simulink model "airplane_pitch_ctrl"  (R2014a)
settings: Solver=ode45  StartTime=0.0  StopTime=5  RelTol=1e-3
libraries: simulink x1
settings Model: Creator=Felix  LastModifiedBy=Felix

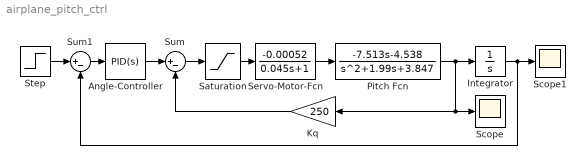
== system airplane_pitch_ctrl ==
  Angle-Controller : simulink/Continuous/PID Controller  Controller=PID  TimeDomain=Continuous-time  SampleTime=1  IntegratorMethod=Forward Euler  FilterMethod=Forward Euler  Form=Parallel  P=7000  I=200  D=1000  N=100  InitialConditionSource=internal  InitialConditionForIntegrator=0  InitialConditionForFilter=0  ExternalReset=none  LimitOutput=off  UpperSaturationLimit=inf  LowerSaturationLimit=-inf  LinearizeAsGain=on  AntiWindupMode=none  Kb=1  TrackingMode=off  Kt=1  PParamMin=[]  PParamMax=[]  PParamDataTypeStr=double  IParamMin=[]  IParamMax=[]  IParamDataTypeStr=double  DParamMin=[]  DParamMax=[]  NParamMin=[]  NParamMax=[]  KbParamMin=[]  KbParamMax=[]  KtParamMin=[]  KtParamMax=[]  POutMin=[]  POutMax=[]  POutDataTypeStr=double  IOutMin=[]  IOutMax=[]  IOutDataTypeStr=double  DOutMin=[]  DOutMax=[]  NOutMin=[]  NOutMax=[]  KbOutMin=[]  KbOutMax=[]  KtOutMin=[]  KtOutMax=[]  IntegratorOutMin=[]  IntegratorOutMax=[]  IntegratorOutDataTypeStr=single  FilterOutMin=[]  FilterOutMax=[]  SumOutMin=[]  SumOutMax=[]  SumOutDataTypeStr=double  SumI1OutMin=[]  SumI1OutMax=[]  SumI2OutMin=[]  SumI2OutMax=[]  SumI3OutMin=[]  SumI3OutMax=[]  SumDOutMin=[]  SumDOutMax=[]  SumAccumDataTypeStr=double  SaturationOutMin=[]  SaturationOutMax=[]  IntegratorContinuousStateAttributes=''  IntegratorStateMustResolveToSignalObject=off  IntegratorRTWStateStorageClass=Auto  FilterContinuousStateAttributes=''  FilterStateMustResolveToSignalObject=off  FilterRTWStateStorageClass=Auto
  Integrator : Integrator
  Kq : Gain  Gain=250
  Pitch Fcn : TransferFcn  Numerator=[-7.513 -4.538]  Denominator=[1 1.99 3.847]
  Saturation : Saturate  UpperLimit=5000  LowerLimit=-5000
  Scope : Scope
  Scope1 : Scope
      settings: TimeRange=1.5  YMin=-1.045075125208682  YMax=-1.031719532554258
  Servo-Motor-Fcn : TransferFcn  Numerator=[-0.00052]  Denominator=[0.045 1]
  Step : Step  Time=0  SampleTime=0
  Sum : Sum  Inputs=|+-
  Sum1 : Sum  Inputs=|+-
  wires:
  Sum1/1 -> Angle-Controller/1
  Pitch Fcn/1 -> Scope/1, Kq/1, Integrator/1
  Integrator/1 -> Sum1/2, Scope1/1
  Kq/1 -> Sum/2
  Servo-Motor-Fcn/1 -> Pitch Fcn/1
  Angle-Controller/1 -> Sum/1
  Step/1 -> Sum1/1
  Saturation/1 -> Servo-Motor-Fcn/1
  Sum/1 -> Saturation/1
